simulink model "s_sswe"  (Simulink 7.8)
settings: Solver=ode4  StartTime=0.0  StopTime=5  FixedStep=0.001  RelTol=1e-3  AbsTol=1e-6
values from neighbouring files (symbols this model uses):
  A = [0 0 1 0 ... (first row only)    [SEESAW_ABCD_eqns.m]
  B = eta_g*Kg*eta_m*Kt/r_mp/Rm*B    [SEESAW_ABCD_eqns.m]
  C = eye(2,4)    [SEESAW_ABCD_eqns.m]
  D = zeros(2,1)    [SEESAW_ABCD_eqns.m]
  K = [ 0 0 0 0 0 ]    [setup_ip02_ssw.m]
  MAX_I_WINDUP = 10 / 180 * pi    (= 0.174532925199)    [setup_ip02_ssw.m]
  MIN_I_WINDUP = - MAX_I_WINDUP    (= -0.174532925199)    [setup_ip02_ssw.m]
  VMAX_AMP = 2.6 * IMAX_AMP    (= 4.16)    [config_ip02.m]
  wcf = 2 * pi * 10    (= 62.8318530718)    [setup_ip02_ssw.m]
  zetaf = 0.9    [setup_ip02_ssw.m]
libraries: simulink_extras x2
settings Model: Creator=MLevis  LastModifiedBy=pmartin  SimulationMode=external  ExtModeTrigDuration=10000  ExtModeAutoUpdateStatusClock=off  BufferReuse=off
settings SolverCC: PositivePriorityOrder=on
settings DataIOCC: LimitDataPoints=off
settings OptimizationCC: BooleanDataType=off  InlineInvariantSignals=on  OptimizeBlockIOStorage=off  BufferReuse=off  ExpressionFolding=off  FoldNonRolledExpr=off  LocalBlockOutputs=off  InitFltsAndDblsToZero=on
settings DebuggingCC: SaveWithParameterizedLinksMsg=none  SignalResolutionControl=TryResolveAllWithWarning  SolverPrmCheckMsg=none  MultiTaskDSMMsg=warning  MultiTaskCondExecSysMsg=none  FcnCallInpInsideContextMsg=Use local settings  StrictBusMsg=None
settings RTWCC: SystemTargetFile=quarc_windows.tlc  TemplateMakefile=quarc_default_tmf  Description=QuaRC Win32 Target  ProcessScript=quarc_windows_make_rtw_hook  IncludeERTFirstTime=on
settings STFCustomTargetCC: TargetFcnLib=ansi_tfl_tmw.mat  TargetPreCompLibLocation=C:\PROGRA~2\QUARC\lib\2011b\windows\release  SystemTargetFile=quarc_windows.tlc
settings GRTTargetCC: TargetFcnLib=ansi_tfl_tmw.mat  TargetPreCompLibLocation=C:\PROGRA~2\QUARC\lib\2011b\windows\release  ParMdlRefBuildCompliant=off  CompOptLevelCompliant=off  ConcurrentExecutionCompliant=off  MatFileLogging=off  ExtMode=on  ExtModeMexFile=quarc_comm

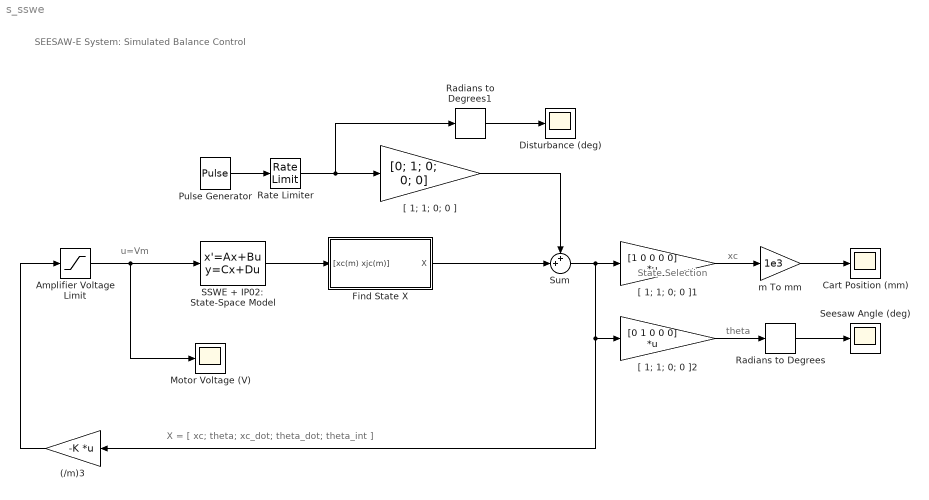
== system s_sswe ==
  note: SEESAW-E System:
      | Simulated Balance Control
  note: u=Vm
  note: X = [ xc; theta; xc_dot; theta_dot; theta_int ]
  note: xc
  note: State Selection
  note: theta
  (/m)3 : Gain  Gain=-K  Multiplication=Matrix(K*u)  SaturateOnIntegerOverflow=on  OutDataTypeStr=Inherit: Same as input  ParamDataTypeStr=Inherit: Same as input
  Amplifier Voltage Limit : Saturate  UpperLimit=VMAX_AMP  LowerLimit=- VMAX_AMP
  Cart Position (mm) : Scope
      settings: TickLabels=on  TimeRange=10  YMin=-200  YMax=200  SaveName=data_xc  DataFormat=Array  MaxDataPoints=10000
  Disturbance (deg) : Scope
      settings: TickLabels=on  TimeRange=10  YMin=-10  YMax=10  SaveName=data_dist  DataFormat=Array  MaxDataPoints=10000
  Find State X : Subsystem
  Motor Voltage (V) : Scope
      settings: TickLabels=on  TimeRange=10  YMin=-11  YMax=8  SaveName=data_vm  DataFormat=Array  MaxDataPoints=10000
  Pulse Generator : DiscretePulseGenerator  PulseType=Time based  Amplitude=0.08  Period=4  PulseWidth=5  PhaseDelay=1
  Radians to Degrees : simulink_extras/Transformations/Radians to Degrees
  Radians to Degrees1 : simulink_extras/Transformations/Radians to Degrees
  Rate Limiter : RateLimiter  RisingSlewLimit=0.5  FallingSlewLimit=-0.5  SampleTimeMode=inherited
  SSWE + IP02: State-Space Model : StateSpace  A=A  B=B  C=C  D=D
  Seesaw Angle (deg) : Scope
      settings: TickLabels=on  TimeRange=10  YMin=-20  YMax=20  SaveName=data_ssw  DataFormat=Array  MaxDataPoints=10000
  Sum : Sum  Inputs=++|
  "[ 1; 1; 0; 0 ]" : Gain  Gain=[0; 1; 0; 0; 0]  SaturateOnIntegerOverflow=on  OutDataTypeStr=Inherit: Same as input  ParamDataTypeStr=Inherit: Same as input
  "[ 1; 1; 0; 0 ]1" : Gain  Gain=[1 0 0 0 0]  Multiplication=Matrix(K*u)  SaturateOnIntegerOverflow=on  OutDataTypeStr=Inherit: Same as input  ParamDataTypeStr=Inherit: Same as input
  "[ 1; 1; 0; 0 ]2" : Gain  Gain=[0 1 0 0 0]  Multiplication=Matrix(K*u)  SaturateOnIntegerOverflow=on  OutDataTypeStr=Inherit: Same as input  ParamDataTypeStr=Inherit: Same as input
  m To mm : Gain  Gain=1e3  SaturateOnIntegerOverflow=on  OutDataTypeStr=Inherit: Same as input  ParamDataTypeStr=Inherit: Same as input
  wires:
  m To mm/1 -> Cart Position (mm)/1
  Radians to Degrees/1 -> Seesaw Angle (deg)/1
  "[ 1; 1; 0; 0 ]2"/1 -> Radians to Degrees/1
  "[ 1; 1; 0; 0 ]1"/1 -> m To mm/1
  (/m)3/1 -> Amplifier Voltage Limit/1
  Amplifier Voltage Limit/1 -> SSWE + IP02: State-Space Model/1, Motor Voltage (V)/1
  Pulse Generator/1 -> Rate Limiter/1
  "[ 1; 1; 0; 0 ]"/1 -> Sum/1
  SSWE + IP02: State-Space Model/1 -> Find State X/1("[xc(m) xjc(m)]")
  Radians to Degrees1/1 -> Disturbance (deg)/1
  Rate Limiter/1 -> "[ 1; 1; 0; 0 ]"/1, Radians to Degrees1/1
  Find State X/1(X) -> Sum/2
  Sum/1 -> "[ 1; 1; 0; 0 ]1"/1, "[ 1; 1; 0; 0 ]2"/1, (/m)3/1

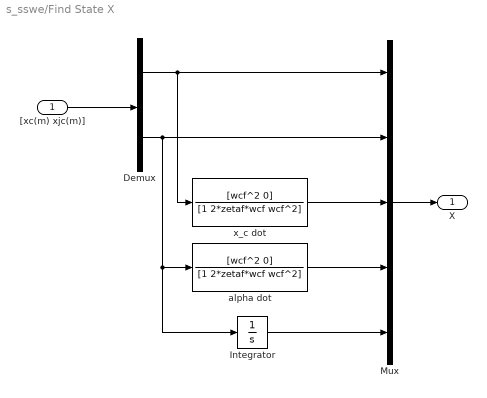
== system s_sswe/Find State X ==
  "[xc(m) xjc(m)]" : Inport
  Demux : Demux  Outputs=2
  Integrator : Integrator  LimitOutput=on  UpperSaturationLimit=MAX_I_WINDUP  LowerSaturationLimit=MIN_I_WINDUP
  Mux : Mux  Inputs=5
  alpha dot : TransferFcn  Numerator=[wcf^2 0]  Denominator=[1 2*zetaf*wcf wcf^2]
  x_c dot : TransferFcn  Numerator=[wcf^2 0]  Denominator=[1 2*zetaf*wcf wcf^2]
  X : Outport  PortDimensions=5
  wires:
  Mux/1 -> X/1
  x_c dot/1 -> Mux/3
  alpha dot/1 -> Mux/4
  "[xc(m) xjc(m)]"/1 -> Demux/1
  Demux/1 -> Mux/1, x_c dot/1
  Demux/2 -> Mux/2, alpha dot/1, Integrator/1
  Integrator/1 -> Mux/5
